simulink model "subscriber_task"  (Simulink 3.0)
libraries: mathlib x1, mqttlib x1, stringlib x1

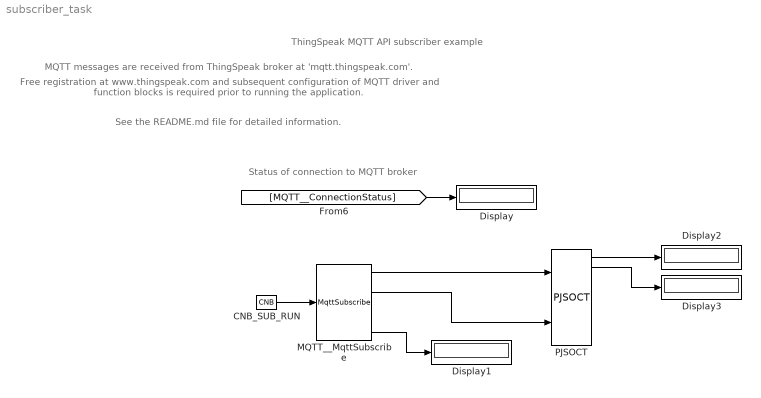
== system subscriber_task ==
  note: Status of connection to MQTT broker
  note: ThingSpeak MQTT API subscriber example
  note: Free registration at www.thingspeak.com and subsequent configuration of MQTT
      | driver and function blocks is required prior to running the application.
  note: See the README.md file for detailed information.
  note: MQTT messages are received from ThingSpeak broker at 'mqtt.thingspeak.com'.
  CNB_SUB_RUN : mathlib/CNB  YCN=on
  Display{,1..3} (4 alike) : Display
      settings: Format=Best fit
  MQTT__MqttSubscribe : mqttlib/MqttSubscribe  topic=channels/<channelID>/subscribe/json/<ReadAPIKey>  QoS=1: QoS0 (At most once)  type=1: string  mode=1: Last value  defBuffSize=2048
  PJSOCT : stringlib/PJSOCT  name1=field1  name2=field2  nmax=0
  wires:
  CNB_SUB_RUN/1 -> MQTT__MqttSubscribe/1
  [MQTT__ConnectionStatus] -> Display/1
  MQTT__MqttSubscribe/1 -> PJSOCT/1
  MQTT__MqttSubscribe/2 -> PJSOCT/2
  MQTT__MqttSubscribe/4 -> Display1/1
  PJSOCT/1 -> Display2/1
  PJSOCT/2 -> Display3/1
